simulink model "pet_hungry"  (R2023a)
settings: Solver=VariableStepAuto  StartTime=0.0  StopTime=24  RelTol=1e-3
settings Model: Creator=laurabryant  LastModifiedBy=laurabryant

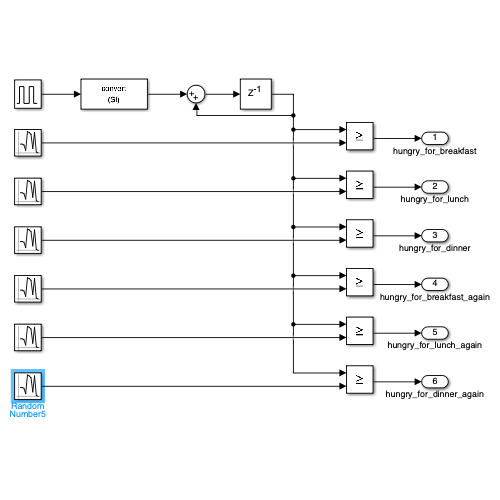
[thumbnail: Simulink's stored preview of the top-level diagram]
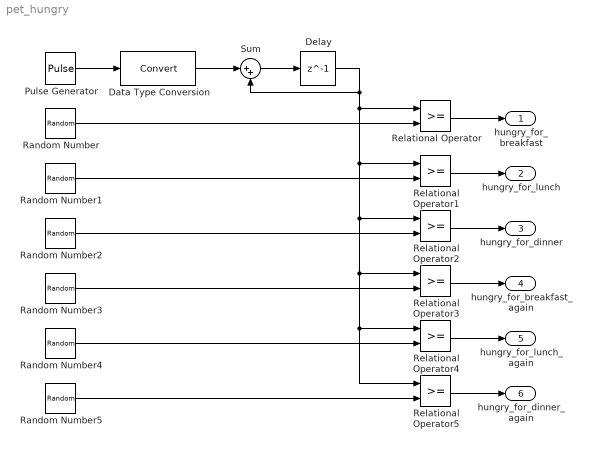
== system pet_hungry ==
  Data Type Conversion : DataTypeConversion  OutMin=0  OutMax=1  ConvertRealWorld=Stored Integer (SI)  RndMeth=Nearest  SaturateOnIntegerOverflow=off
  Delay : Delay  DelayLength=1  InitialCondition=0  SampleTime=1
  Pulse Generator : DiscretePulseGenerator  PulseType=Time based  Period=1  PulseWidth=5
  Random Number : RandomNumber  Mean=4  Variance=2  SampleTime=48
  Random Number1 : RandomNumber  Mean=10  Variance=2  Seed=1  SampleTime=48
  Random Number2 : RandomNumber  Mean=20  Variance=2  Seed=2  SampleTime=48
  Random Number3 : RandomNumber  Mean=28  Variance=2  Seed=3  SampleTime=48
  Random Number4 : RandomNumber  Mean=36  Variance=2  Seed=4  SampleTime=48
  Random Number5 : RandomNumber  Mean=44  Variance=2  Seed=5  SampleTime=48
  Relational Operator{,1..5} (6 alike) : RelationalOperator  OutDataTypeStr=boolean  RndMeth=Simplest  InputSameDT=off
  Sum : Sum  Inputs=|++
  hungry_for_breakfast : Outport
  hungry_for_lunch : Outport  Port=2
  hungry_for_dinner : Outport  Port=3
  hungry_for_breakfast_again : Outport  Port=4
  hungry_for_lunch_again : Outport  Port=5
  hungry_for_dinner_again : Outport  Port=6
  wires:
  Pulse Generator/1 -> Data Type Conversion/1
  Data Type Conversion/1 -> Sum/1
  Sum/1 -> Delay/1
  Random Number/1 -> Relational Operator/2
  Relational Operator/1 -> hungry_for_breakfast/1
  Relational Operator1/1 -> hungry_for_lunch/1
  Random Number1/1 -> Relational Operator1/2
  Relational Operator2/1 -> hungry_for_dinner/1
  Random Number2/1 -> Relational Operator2/2
  Relational Operator3/1 -> hungry_for_breakfast_again/1
  Random Number3/1 -> Relational Operator3/2
  Relational Operator4/1 -> hungry_for_lunch_again/1
  Random Number4/1 -> Relational Operator4/2
  Delay/1 -> Relational Operator/1, Relational Operator5/1, Relational Operator4/1, Relational Operator3/1, Relational Operator2/1, Relational Operator1/1, Sum/2
  Relational Operator5/1 -> hungry_for_dinner_again/1
  Random Number5/1 -> Relational Operator5/2
